simulink model "modelo_cinematico_directo"  (R2015a)
settings: Solver=ode45  StartTime=0.0  StopTime=50  RelTol=1e-3
settings Model: Creator=samir  LastModifiedBy=samir

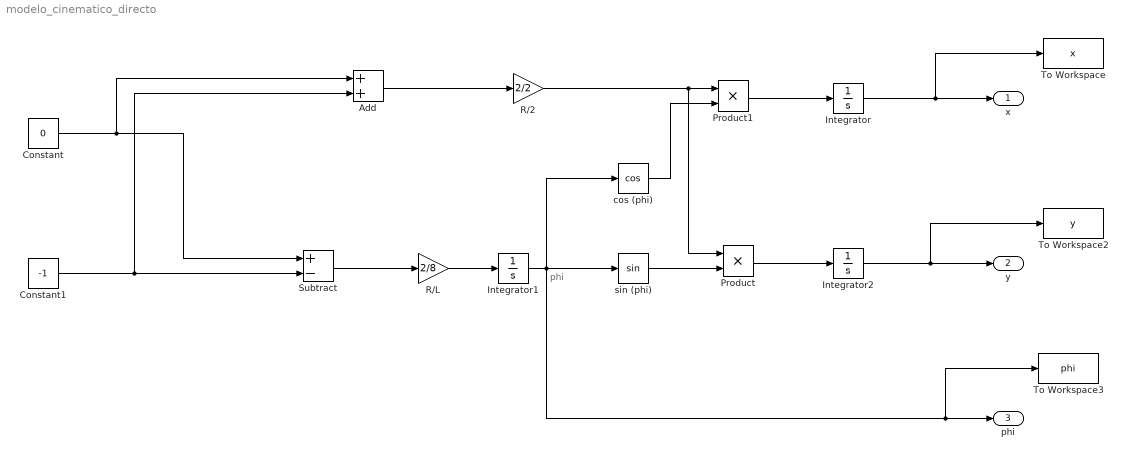
== system modelo_cinematico_directo ==
  note: phi
  Add : Sum
  Constant : Constant  Value=0
  Constant1 : Constant  Value=-1
  Integrator : Integrator
  Integrator1 : Integrator
  Integrator2 : Integrator
  Product : Product
  Product1 : Product
  R/2 : Gain  Gain=2/2
  R/L : Gain  Gain=2/8
  Subtract : Sum  Inputs=+-
  To Workspace : ToWorkspace  VariableName=x  SaveFormat=Timeseries  SampleTime=-1
  To Workspace2 : ToWorkspace  VariableName=y  SaveFormat=Timeseries  SampleTime=-1
  To Workspace3 : ToWorkspace  VariableName=phi  SaveFormat=Timeseries  SampleTime=-1
  cos (phi) : Trigonometry  Operator=cos
  sin (phi) : Trigonometry
  x : Outport
  y : Outport  Port=2
  phi : Outport  Port=3
  wires:
  Constant1/1 -> Add/2, Subtract/2
  Constant/1 -> Add/1, Subtract/1
  Subtract/1 -> R/L/1
  R/L/1 -> Integrator1/1
  Integrator1/1 -> To Workspace3/1, phi/1, cos (phi)/1, sin (phi)/1
  Add/1 -> R/2/1
  R/2/1 -> Product/1, Product1/1
  cos (phi)/1 -> Product1/2
  sin (phi)/1 -> Product/2
  Product1/1 -> Integrator/1
  Product/1 -> Integrator2/1
  Integrator/1 -> To Workspace/1, x/1
  Integrator2/1 -> To Workspace2/1, y/1
